simulink model "statetest"  (Simulink 3.00)
settings: Solver=ode23tb  StartTime=0.0  StopTime=10  RelTol=1e-3
values from neighbouring files (symbols this model uses):
  D = [i1 20e-3 11.4e-3  31.76e-3 2 ... (first row only)    [lacm2.m]    (also in lacm3.m; lacm4a.m; lacm4b.m; lacm4c.m)
undefined symbols (not defined in the file or in its folder): A, B, C

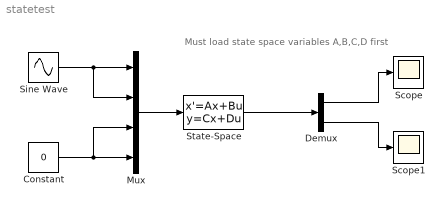
== system statetest ==
  note: Must load state space variables A,B,C,D first
  Constant : Constant  Value=0
  Demux : Demux  Outputs=2
  Mux : Mux  Inputs=4
  Scope : Scope
      settings: TimeRange=auto  YMin=-1  YMax=1  SaveToWorkspace=off  SaveName=ScopeData
  Scope1 : Scope
      settings: TimeRange=auto  YMin=-1  YMax=1  SaveToWorkspace=off  SaveName=ScopeData
  Sine Wave : Sin  Amplitude=200  Frequency=2*pi  Phase=0  SampleTime=0
  State-Space : StateSpace  A=A  B=B  C=C  D=D  X0=0
  wires:
  Mux/1 -> State-Space/1
  State-Space/1 -> Demux/1
  Demux/1 -> Scope/1
  Demux/2 -> Scope1/1
  Sine Wave/1 -> Mux/1, Mux/2
  Constant/1 -> Mux/4, Mux/3
